simulink model "RandomPhaseMultisine"  (R2019b)
settings: Solver=VariableStepAuto  StartTime=0.0  StopTime=10.0  RelTol=1e-3
libraries: simulink x1
settings Model: Creator=s164234  LastModifiedBy=s164234

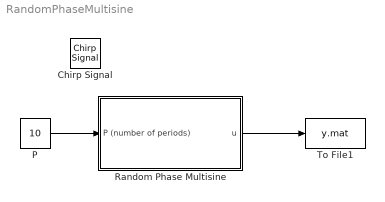
== system RandomPhaseMultisine ==
  Chirp Signal : simulink/Sources/Chirp Signal  f1=0.1  T=100  f2=1
  P : Constant  Value=10  SampleTime=0.001
  "Random Phase Multisine " : Subsystem
  To File1 : ToFile  Filename=y.mat  MatrixName=y  SaveFormat=Timeseries  SampleTime=0.001
  wires:
  P/1 -> "Random Phase Multisine "/1("P (number of periods) ")
  "Random Phase Multisine "/1(u) -> To File1/1

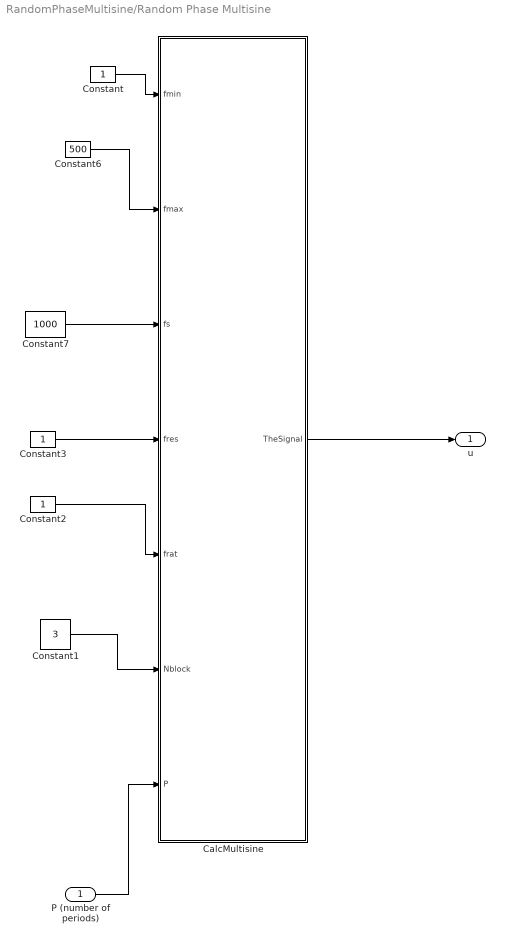
== system RandomPhaseMultisine/Random Phase Multisine  ==
  "P (number of periods) " : Inport
  "CalcMultisine " : MATLAB Function  TreatAsAtomicUnit=on  SystemSampleTime=0.001
  Constant : Constant
  Constant1 : Constant  Value=3
  Constant2 : Constant
  Constant3 : Constant
  Constant6 : Constant  Value=500
  Constant7 : Constant  Value=1000
  u : Outport  PortDimensions=1  SampleTime=0.001
  wires:
  "CalcMultisine "/1(TheSignal) -> u/1
  "P (number of periods) "/1 -> "CalcMultisine "/7(P)
  Constant/1 -> "CalcMultisine "/1(fmin)
  Constant6/1 -> "CalcMultisine "/2(fmax)
  Constant7/1 -> "CalcMultisine "/3(fs)
  Constant2/1 -> "CalcMultisine "/5(frat)
  Constant1/1 -> "CalcMultisine "/6(Nblock)
  Constant3/1 -> "CalcMultisine "/4(fres)

== matlab function RandomPhaseMultisine/Random Phase Multisine /CalcMultisine  ==
  settings: updateMethod=DISCRETE  sampleTime=0.001
  data: fmin input; fmax input; fs input; fres input; frat input; Nblock input; TheSignal output size=1; P input
function TheSignal = CalcMultisine(fmin, fmax, fs, fres, frat, Nblock, P)

ExcitedHarm = [2,3,5,6,8,9,11,12,14,15,17,18,20,21,23,24,26,27,29,30,32,33,35,36,38,39,41,42,44,45,47,48,50,51,53,54,56,57,59,60,62,63,65,66,68,69,71,72,74,75,77,78,80,81,83,84,86,87,89,90,92,93,95,96,98,99,101,102,104,105,107,108,110,111,113,114,116,117,119,120,122,123,125,126,128,129,131,132,134,135,137,138,140,141,143,144,146,147,149,150,152,153,155,156,158,159,161,162,164,165,167,168,170,171,173,174,176,177,179,180,182,183,185,186,188,189,191,192,194,195,197,198,200,201,203,204,206,207,209,210,212,213,215,216,218,219,221,222,224,225,227,228,230,231,233,234,236,237,239,240,242,243,245,246,248,249,251,252,254,255,257,258,260,261,263,264,266,267,269,270,272,273,275,276,278,279,281,282,284,285,287,288,290,291,293,294,296,297,299,300,302,303,305,306,308,309,311,312,314,315,317,318,320,321,323,324,326,327,329,330,332,333,335,336,338,339,341,342,344,345,347,348,350,351,353,354,356,357,359,360,362,363,365,366,368,369,371,372,374,375,377,378,380,381,383,384,386,387,389,390,392,393,395,396,398,399,401,402,404,405,407,408,410,411,413,414,416,417,419,420,422,423,425,426,428,429,431,432,434,435,437,438,440,441,443,444,446,447,449,450,452,453,455,456,458,459,461,462,464,465,467,468,470,471,473,474,476,477,479,480,482,483,485,486,488,489,491,492,494,495,497,498,500];

N = ceil(fs/fres);                  % number of time domain points in one period
fres = fs/N;
FreqSpan = floor(fmax/fres);        % frequency span for a lowpass signal

TheSignal = zeros(10000,1);

a = zeros(1000,1);
b = zeros(1000,1);

S = complex(a,b);

%S = zeros(1000,1);

S(ExcitedHarm + 1) = ones(size(ExcitedHarm)) .* exp(i*2*pi*rand(size(ExcitedHarm)));
u = 2*real(ifft(S));

TheSignal = repmat(u,10,1);
